simulink model "GuytonModel1986All_R2015a"  (R2015a)
settings: Solver=ode15s  StartTime=0  StopTime=383040  FixedStep=0.03  MaxStep=360  RelTol=1e-3
libraries: simulink x3
(part 5 of 5)

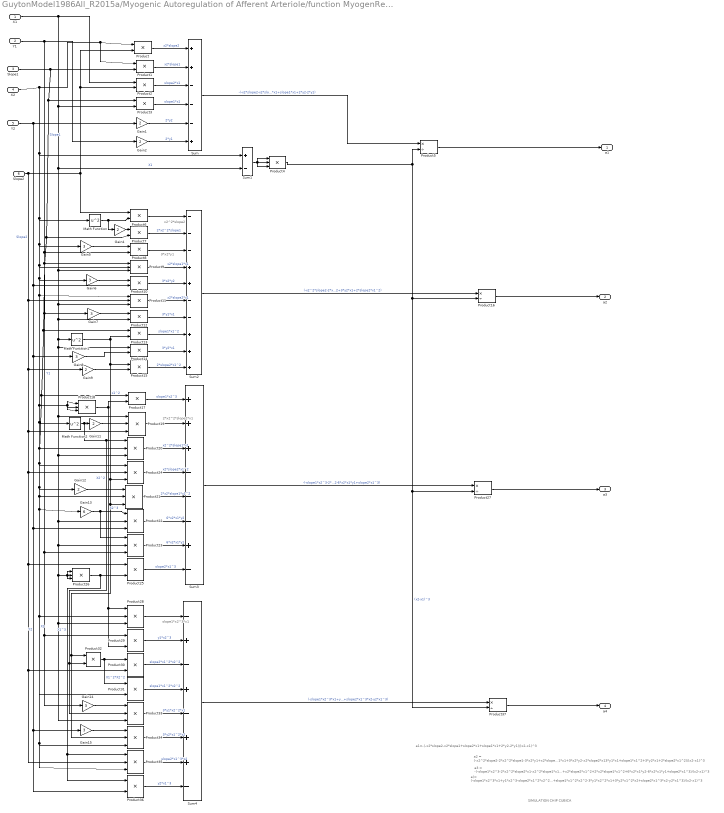
== system GuytonModel1986All_R2015a/Myogenic Autoregulation of Afferent Arteriole/function MyogenResp(PDIFF) - spline interpolation/If Action Subsystem/Cubica ==
  note: SIMULATION CHIP CUBICA
  note: a)= (-slope1*x2^3*x1+y1*x2^3-slope2*x1^2*x2^2+slope1*x1^2*x2^2-3*y1*x2^2*x1+3*y2*x1^2*x2+slope2*x1^3*x2-y2*x1^3)/(x2-x1)^3
  note: a3 = -(-slope1*x2^3-2*x2^2*slope2*x1-x2^2*slope1*x1+x2*slope2*x1^2+2*x2*slope1*x1^2+6*x2*x1*y2-6*x2*x1*y1+slope2*x1^3)/(x2-x1)^3
  note: a2 = (-x2^2*slope2-2*x2^2*slope1-3*x2*y1+x2*slope1*x1+3*x2*y2-x2*slope2*x13*y1*x1+slope1*x1^2+3*y2*x1+2*slope2*x1^2)/(x2-x1)^3
  note: slope1*x2^3*x1
  note: 2*x2^2*slope2*x1
  note: 3*x2*y1
  note: x2^2*slope2
  note: a1=-(-x2*slope2-x2*slope1+slope2*x1+slope1*x1+2*y2-2*y1)/(x2-x1)^3
  X1 : Inport
  Y1 : Inport  Port=2
  Slope1 : Inport  Port=3
  X2 : Inport  Port=4
  Y2 : Inport  Port=5
  Slope2 : Inport  Port=6
  Gain{1..2,4,9,11..12} (6 alike) : Gain  Gain=2  SaturateOnIntegerOverflow=on  OutDataTypeStr=Inherit: Same as input  ParamDataTypeStr=Inherit: Same as input
  Gain13 : Gain  Gain=6  SaturateOnIntegerOverflow=on  OutDataTypeStr=Inherit: Same as input  ParamDataTypeStr=Inherit: Same as input
  Gain{5..8,14..15} (6 alike) : Gain  Gain=3  SaturateOnIntegerOverflow=on  OutDataTypeStr=Inherit: Same as input  ParamDataTypeStr=Inherit: Same as input
  Math Function : Math  Operator=square  SaturateOnIntegerOverflow=on
  Math Function1 : Math  Operator=square  SaturateOnIntegerOverflow=on
  Math Function2 : Math  Operator=square  SaturateOnIntegerOverflow=on
  Product{,1..3,6..8,10,12..15,17,25,29..32,36} (19 alike) : Product  SaturateOnIntegerOverflow=on  InputSameDT=on  OutDataTypeStr=Inherit: Same as first input
  Product{4,9,11,18..24,26,28,33..35} (15 alike) : Product  Inputs=3  SaturateOnIntegerOverflow=on  InputSameDT=on  OutDataTypeStr=Inherit: Same as first input
  Product{5,16,27,37} (4 alike) : Product  Inputs=*/  SaturateOnIntegerOverflow=on  InputSameDT=on  OutDataTypeStr=Inherit: Same as first input
  Sum : Sum  Inputs=++---+  SaturateOnIntegerOverflow=on  InputSameDT=on  OutDataTypeStr=Inherit: Same as first input
  Sum1 : Sum  Inputs=+-  SaturateOnIntegerOverflow=on  InputSameDT=on  OutDataTypeStr=Inherit: Same as first input
  Sum2 : Sum  Inputs=---++--+++  SaturateOnIntegerOverflow=on  InputSameDT=on  OutDataTypeStr=Inherit: Same as first input
  Sum3 : Sum  Inputs=+++---+-  SaturateOnIntegerOverflow=on  InputSameDT=on  OutDataTypeStr=Inherit: Same as first input
  Sum4 : Sum  Inputs=-+-+-++-  SaturateOnIntegerOverflow=on  InputSameDT=on  OutDataTypeStr=Inherit: Same as first input
  a1 : Outport
  a2 : Outport  Port=2
  a3 : Outport  Port=3
  a4 : Outport  Port=4
  wires:
  Sum3/1 -> Product27/1  "-(-slope1*x2^3-2*x2^2*slope2*x1-x2^2*slope1*x1+x2*slope2*x1^2+2*x2*slope1*x1^2+6*x2*x1*y2-6*x2*x1*y1+slope2*x1^3)"
  Product37/1 -> a4/1
  Sum4/1 -> Product37/1  "(-slope1*x2^3*x1+y1*x2^3-slope2*x1^2*x2^2+slope1*x1^2*x2^2-3*y1*x2^2*x1+3*y2*x1^2*x2+slope2*x1^3*x2-y2*x1^3)"
  Product36/1 -> Sum4/8  "y2*x1^3"
  Product35/1 -> Sum4/7  "slope2*x1^3*x2"
  Gain15/1 -> Product34/1
  Product34/1 -> Sum4/6  "3*y2*x1^2*x2"
  Gain14/1 -> Product33/1
  Product33/1 -> Sum4/5  "3*y1*x2^2*x1"
  Product32/1 -> Product31/1, Product30/1  "X1^2*X2^2"
  Product31/1 -> Sum4/4  "slope1*x1^2*x2^2"
  Product30/1 -> Sum4/3  "slope2*x1^2*x2^2"
  Product29/1 -> Sum4/2  "y1*x2^3"
  Product28/1 -> Sum4/1
  Product27/1 -> a3/1
  Product26/1 -> Product36/1, Product35/1, Product25/2  "X1^3"
  Product25/1 -> Sum3/8  "slope2*x1^3"
  Product24/1 -> Sum3/4  "x2*slope2*x1^2"
  Product21/1 -> Sum3/5  "2*x2*slope1*x1^2"
  Product22/1 -> Sum3/6  "6*x2*x1*y2"
  Product23/1 -> Sum3/7  "6*x2*x1*y1"
  Gain13/1 -> Product23/1, Product22/1
  Gain12/1 -> Product21/1
  Product20/1 -> Sum3/3  "x2^2*slope1*x1"
  Gain11/1 -> Product19/2
  Math Function2/1 -> Product33/2, Product32/2, Product20/1, Gain11/1  "X2^2"
  Product19/1 -> Sum3/2
  Product18/1 -> Product29/2, Product28/1, Product17/2  "X2^3"
  Product17/1 -> Sum3/1  "slope1*x2^3"
  Product16/1 -> a2/1
  Sum2/1 -> Product16/1  "(-x2^2*slope2-2*x2^2*slope1-3*x2*y1+x2*slope1*x1+3*x2*y2-x2*slope2*x1-3*y1*x1+slope1*x1^2+3*y2*x1+2*slope2*x1^2)"
  Gain9/1 -> Product15/2
  Product15/1 -> Sum2/10  "2*slope2*x1^2"
  Gain8/1 -> Product14/2
  Product14/1 -> Sum2/9  "3*y2*x1"
  Math Function1/1 -> Product34/2, Product32/1, Product21/3, Product24/3, Product15/1, Product13/2  "x1^2"
  Product13/1 -> Sum2/8  "slope1*x1^2"
  Gain7/1 -> Product12/1
  Product12/1 -> Sum2/7  "3*y1*x1"
  Product11/1 -> Sum2/6  "x2*slope2*x1"
  Product10/1 -> Sum2/5  "3*x2*y2"
  Gain6/1 -> Product10/1
  Product9/1 -> Sum2/4  "x2*slope1*x1"
  Gain5/1 -> Product8/1
  Product8/1 -> Sum2/3
  Product7/1 -> Sum2/2  "2*x2^2*slope1"
  Gain4/1 -> Product7/1
  Product6/1 -> Sum2/1
  Math Function/1 -> Gain4/1, Product6/2
  Product5/1 -> a1/1
  Product4/1 -> Product37/2, Product27/2, Product16/2, Product5/2  "(x2-x1)^3"
  Sum1/1 -> Product4/1, Product4/3, Product4/2
  Sum/1 -> Product5/1  "-(-x2*slope2-x2*slope1+slope2*x1+slope1*x1+2*y2-2*y1)"
  Y1/1 -> Gain14/1, Product29/1, Product23/3, Gain7/1, Product8/2, Gain2/1  "Y1"
  Gain2/1 -> Sum/6  "2*y1"
  Gain1/1 -> Sum/5  "2*y2"
  Y2/1 -> Product36/2, Gain15/1, Product22/3, Gain8/1, Product10/2, Gain1/1  "Y2"
  Product3/1 -> Sum/4  "slope1*x1"
  Product2/1 -> Sum/3  "slope2*x1"
  X1/1 -> Sum1/2, Product33/3, Product28/3, Product26/1, Product26/3, Product26/2, Product23/2, Product22/2, Product20/3, Product19/1, Product14/1, Math Function1/1, Product12/2, Product11/3, Product9/3, Product3/2, Product2/1  "X1"
  Product1/1 -> Sum/2  "x2*slope1"
  Product/1 -> Sum/1  "x2*slope2"
  Slope1/1 -> Product31/2, Product28/2, Product21/2, Product20/2, Product17/1, Product13/1, Product9/1, Product7/2, Product3/1, Product1/2  "Slope1"
  Slope2/1 -> Product35/2, Product30/2, Product25/1, Product24/2, Product19/3, Gain9/1, Product11/2, Product6/1, Product2/2, Product/2  "Slope2"
  X2/1 -> Product/1, Product1/1, Product24/1, Product35/3, Product34/3, Gain13/1, Gain12/1, Math Function2/1, Product18/3, Product18/1, Product18/2, Product11/1, Gain6/1, Product9/2, Gain5/1, Math Function/1, Sum1/1  "X2"

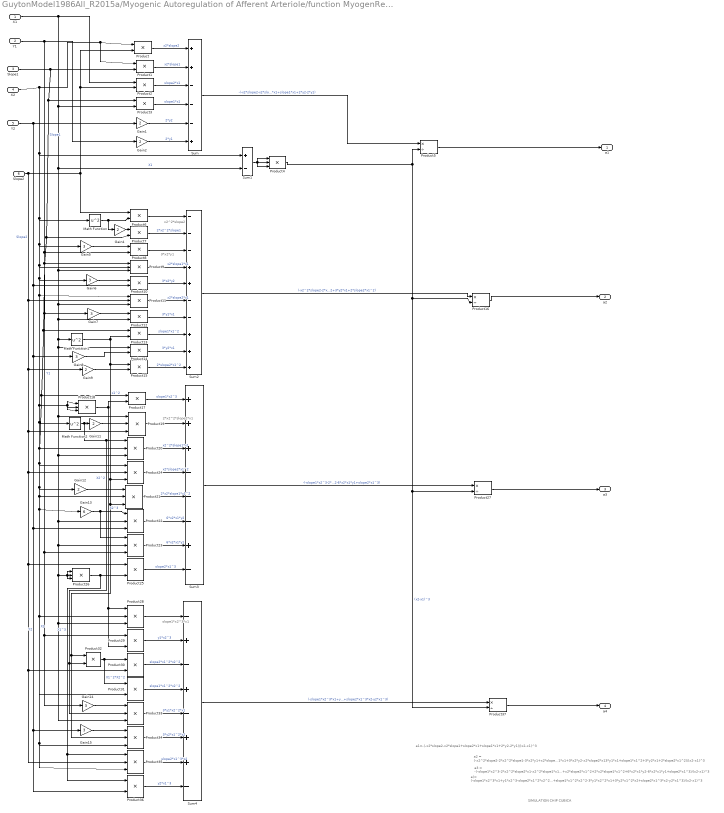
== system GuytonModel1986All_R2015a/Myogenic Autoregulation of Afferent Arteriole/function MyogenResp(PDIFF) - spline interpolation/If Action Subsystem/Cubica1 ==
  note: SIMULATION CHIP CUBICA
  note: a)= (-slope1*x2^3*x1+y1*x2^3-slope2*x1^2*x2^2+slope1*x1^2*x2^2-3*y1*x2^2*x1+3*y2*x1^2*x2+slope2*x1^3*x2-y2*x1^3)/(x2-x1)^3
  note: a3 = -(-slope1*x2^3-2*x2^2*slope2*x1-x2^2*slope1*x1+x2*slope2*x1^2+2*x2*slope1*x1^2+6*x2*x1*y2-6*x2*x1*y1+slope2*x1^3)/(x2-x1)^3
  note: a2 = (-x2^2*slope2-2*x2^2*slope1-3*x2*y1+x2*slope1*x1+3*x2*y2-x2*slope2*x13*y1*x1+slope1*x1^2+3*y2*x1+2*slope2*x1^2)/(x2-x1)^3
  note: slope1*x2^3*x1
  note: 2*x2^2*slope2*x1
  note: 3*x2*y1
  note: x2^2*slope2
  note: a1=-(-x2*slope2-x2*slope1+slope2*x1+slope1*x1+2*y2-2*y1)/(x2-x1)^3
  X1 : Inport
  Y1 : Inport  Port=2
  Slope1 : Inport  Port=3
  X2 : Inport  Port=4
  Y2 : Inport  Port=5
  Slope2 : Inport  Port=6
  Gain{1..2,4,9,11..12} (6 alike) : Gain  Gain=2  SaturateOnIntegerOverflow=on  OutDataTypeStr=Inherit: Same as input  ParamDataTypeStr=Inherit: Same as input
  Gain13 : Gain  Gain=6  SaturateOnIntegerOverflow=on  OutDataTypeStr=Inherit: Same as input  ParamDataTypeStr=Inherit: Same as input
  Gain{5..8,14..15} (6 alike) : Gain  Gain=3  SaturateOnIntegerOverflow=on  OutDataTypeStr=Inherit: Same as input  ParamDataTypeStr=Inherit: Same as input
  Math Function : Math  Operator=square  SaturateOnIntegerOverflow=on
  Math Function1 : Math  Operator=square  SaturateOnIntegerOverflow=on
  Math Function2 : Math  Operator=square  SaturateOnIntegerOverflow=on
  Product{,1..3,6..8,10,12..15,17,25,29..32,36} (19 alike) : Product  SaturateOnIntegerOverflow=on  InputSameDT=on  OutDataTypeStr=Inherit: Same as first input
  Product{4,9,11,18..24,26,28,33..35} (15 alike) : Product  Inputs=3  SaturateOnIntegerOverflow=on  InputSameDT=on  OutDataTypeStr=Inherit: Same as first input
  Product{5,16,27,37} (4 alike) : Product  Inputs=*/  SaturateOnIntegerOverflow=on  InputSameDT=on  OutDataTypeStr=Inherit: Same as first input
  Sum : Sum  Inputs=++---+  SaturateOnIntegerOverflow=on  InputSameDT=on  OutDataTypeStr=Inherit: Same as first input
  Sum1 : Sum  Inputs=+-  SaturateOnIntegerOverflow=on  InputSameDT=on  OutDataTypeStr=Inherit: Same as first input
  Sum2 : Sum  Inputs=---++--+++  SaturateOnIntegerOverflow=on  InputSameDT=on  OutDataTypeStr=Inherit: Same as first input
  Sum3 : Sum  Inputs=+++---+-  SaturateOnIntegerOverflow=on  InputSameDT=on  OutDataTypeStr=Inherit: Same as first input
  Sum4 : Sum  Inputs=-+-+-++-  SaturateOnIntegerOverflow=on  InputSameDT=on  OutDataTypeStr=Inherit: Same as first input
  a1 : Outport
  a2 : Outport  Port=2
  a3 : Outport  Port=3
  a4 : Outport  Port=4
  wires:
  Sum3/1 -> Product27/1  "-(-slope1*x2^3-2*x2^2*slope2*x1-x2^2*slope1*x1+x2*slope2*x1^2+2*x2*slope1*x1^2+6*x2*x1*y2-6*x2*x1*y1+slope2*x1^3)"
  Product37/1 -> a4/1
  Sum4/1 -> Product37/1  "(-slope1*x2^3*x1+y1*x2^3-slope2*x1^2*x2^2+slope1*x1^2*x2^2-3*y1*x2^2*x1+3*y2*x1^2*x2+slope2*x1^3*x2-y2*x1^3)"
  Product36/1 -> Sum4/8  "y2*x1^3"
  Product35/1 -> Sum4/7  "slope2*x1^3*x2"
  Gain15/1 -> Product34/1
  Product34/1 -> Sum4/6  "3*y2*x1^2*x2"
  Gain14/1 -> Product33/1
  Product33/1 -> Sum4/5  "3*y1*x2^2*x1"
  Product32/1 -> Product31/1, Product30/1  "X1^2*X2^2"
  Product31/1 -> Sum4/4  "slope1*x1^2*x2^2"
  Product30/1 -> Sum4/3  "slope2*x1^2*x2^2"
  Product29/1 -> Sum4/2  "y1*x2^3"
  Product28/1 -> Sum4/1
  Product27/1 -> a3/1
  Product26/1 -> Product36/1, Product35/1, Product25/2  "X1^3"
  Product25/1 -> Sum3/8  "slope2*x1^3"
  Product24/1 -> Sum3/4  "x2*slope2*x1^2"
  Product21/1 -> Sum3/5  "2*x2*slope1*x1^2"
  Product22/1 -> Sum3/6  "6*x2*x1*y2"
  Product23/1 -> Sum3/7  "6*x2*x1*y1"
  Gain13/1 -> Product23/1, Product22/1
  Gain12/1 -> Product21/1
  Product20/1 -> Sum3/3  "x2^2*slope1*x1"
  Gain11/1 -> Product19/2
  Math Function2/1 -> Product33/2, Product32/2, Product20/1, Gain11/1  "X2^2"
  Product19/1 -> Sum3/2
  Product18/1 -> Product29/2, Product28/1, Product17/2  "X2^3"
  Product17/1 -> Sum3/1  "slope1*x2^3"
  Product16/1 -> a2/1
  Sum2/1 -> Product16/1  "(-x2^2*slope2-2*x2^2*slope1-3*x2*y1+x2*slope1*x1+3*x2*y2-x2*slope2*x1-3*y1*x1+slope1*x1^2+3*y2*x1+2*slope2*x1^2)"
  Gain9/1 -> Product15/2
  Product15/1 -> Sum2/10  "2*slope2*x1^2"
  Gain8/1 -> Product14/2
  Product14/1 -> Sum2/9  "3*y2*x1"
  Math Function1/1 -> Product34/2, Product32/1, Product21/3, Product24/3, Product15/1, Product13/2  "x1^2"
  Product13/1 -> Sum2/8  "slope1*x1^2"
  Gain7/1 -> Product12/1
  Product12/1 -> Sum2/7  "3*y1*x1"
  Product11/1 -> Sum2/6  "x2*slope2*x1"
  Product10/1 -> Sum2/5  "3*x2*y2"
  Gain6/1 -> Product10/1
  Product9/1 -> Sum2/4  "x2*slope1*x1"
  Gain5/1 -> Product8/1
  Product8/1 -> Sum2/3
  Product7/1 -> Sum2/2  "2*x2^2*slope1"
  Gain4/1 -> Product7/1
  Product6/1 -> Sum2/1
  Math Function/1 -> Gain4/1, Product6/2
  Product5/1 -> a1/1
  Product4/1 -> Product37/2, Product27/2, Product16/2, Product5/2  "(x2-x1)^3"
  Sum1/1 -> Product4/1, Product4/3, Product4/2
  Sum/1 -> Product5/1  "-(-x2*slope2-x2*slope1+slope2*x1+slope1*x1+2*y2-2*y1)"
  Y1/1 -> Gain14/1, Product29/1, Product23/3, Gain7/1, Product8/2, Gain2/1  "Y1"
  Gain2/1 -> Sum/6  "2*y1"
  Gain1/1 -> Sum/5  "2*y2"
  Y2/1 -> Product36/2, Gain15/1, Product22/3, Gain8/1, Product10/2, Gain1/1  "Y2"
  Product3/1 -> Sum/4  "slope1*x1"
  Product2/1 -> Sum/3  "slope2*x1"
  X1/1 -> Sum1/2, Product33/3, Product28/3, Product26/1, Product26/3, Product26/2, Product23/2, Product22/2, Product20/3, Product19/1, Product14/1, Math Function1/1, Product12/2, Product11/3, Product9/3, Product3/2, Product2/1  "X1"
  Product1/1 -> Sum/2  "x2*slope1"
  Product/1 -> Sum/1  "x2*slope2"
  Slope1/1 -> Product31/2, Product28/2, Product21/2, Product20/2, Product17/1, Product13/1, Product9/1, Product7/2, Product3/1, Product1/2  "Slope1"
  Slope2/1 -> Product35/2, Product30/2, Product25/1, Product24/2, Product19/3, Gain9/1, Product11/2, Product6/1, Product2/2, Product/2  "Slope2"
  X2/1 -> Product/1, Product1/1, Product24/1, Product35/3, Product34/3, Gain13/1, Gain12/1, Math Function2/1, Product18/3, Product18/1, Product18/2, Product11/1, Gain6/1, Product9/2, Gain5/1, Math Function/1, Sum1/1  "X2"

== system GuytonModel1986All_R2015a/Myogenic Autoregulation of Afferent Arteriole/function MyogenResp(PDIFF) - spline interpolation/Subsystem/If Action Subsystem ==
  x : Inport
  aa4 : Inport  Port=2
  "aa6 " : Inport  Port=3
  Action Port : ActionPort  ActionType=then
  Product : Product  SaturateOnIntegerOverflow=on  InputSameDT=on  OutDataTypeStr=Inherit: Same as first input
  Sum : Sum  SaturateOnIntegerOverflow=on  InputSameDT=on  OutDataTypeStr=Inherit: Same as first input
  y : Outport
  wires:
  Sum/1 -> y/1  "y=aa4*x+aa5"
  "aa6 "/1 -> Sum/2
  Product/1 -> Sum/1
  x/1 -> Product/1
  aa4/1 -> Product/2

== system GuytonModel1986All_R2015a/Myogenic Autoregulation of Afferent Arteriole/function MyogenResp(PDIFF) - spline interpolation/Subsystem/If Action Subsystem1 ==
  x : Inport
  aa6 : Inport  Port=2
  aa7 : Inport  Port=3
  aa8 : Inport  Port=4
  aa9 : Inport  Port=5
  Action Port : ActionPort  ActionType=elseif
  Math Function : Math  Operator=square  SaturateOnIntegerOverflow=on
  Product : Product  Inputs=3  SaturateOnIntegerOverflow=on  InputSameDT=on  OutDataTypeStr=Inherit: Same as first input
  Product2 : Product  SaturateOnIntegerOverflow=on  InputSameDT=on  OutDataTypeStr=Inherit: Same as first input
  Product3 : Product  SaturateOnIntegerOverflow=on  InputSameDT=on  OutDataTypeStr=Inherit: Same as first input
  Sum : Sum  Inputs=++++  SaturateOnIntegerOverflow=on  InputSameDT=on  OutDataTypeStr=Inherit: Same as first input
  y : Outport
  wires:
  Sum/1 -> y/1  "y=aa6*x^3+aa7*x^2+aa8*x+aa9"
  aa9/1 -> Sum/4
  Product3/1 -> Sum/3
  aa8/1 -> Product3/2
  Product2/1 -> Sum/2
  aa7/1 -> Product2/2
  aa6/1 -> Product/3
  Product/1 -> Sum/1
  Math Function/1 -> Product2/1, Product/1
  x/1 -> Product3/1, Product/2, Math Function/1

== system GuytonModel1986All_R2015a/Myogenic Autoregulation of Afferent Arteriole/function MyogenResp(PDIFF) - spline interpolation/Subsystem/If Action Subsystem2 ==
  x : Inport
  aa10 : Inport  Port=2
  aa11 : Inport  Port=3
  aa12 : Inport  Port=4
  aa13 : Inport  Port=5
  Action Port : ActionPort  ActionType=elseif
  Math Function : Math  Operator=square  SaturateOnIntegerOverflow=on
  Product : Product  Inputs=3  SaturateOnIntegerOverflow=on  InputSameDT=on  OutDataTypeStr=Inherit: Same as first input
  Product2 : Product  SaturateOnIntegerOverflow=on  InputSameDT=on  OutDataTypeStr=Inherit: Same as first input
  Product3 : Product  SaturateOnIntegerOverflow=on  InputSameDT=on  OutDataTypeStr=Inherit: Same as first input
  Sum : Sum  Inputs=++++  SaturateOnIntegerOverflow=on  InputSameDT=on  OutDataTypeStr=Inherit: Same as first input
  y : Outport
  wires:
  x/1 -> Math Function/1, Product/2, Product3/1
  Math Function/1 -> Product/1, Product2/1
  Product/1 -> Sum/1
  aa10/1 -> Product/3
  aa11/1 -> Product2/2
  Product2/1 -> Sum/2
  aa12/1 -> Product3/2
  Product3/1 -> Sum/3
  aa13/1 -> Sum/4
  Sum/1 -> y/1  "y=aa6*x^3+aa7*x^2+aa8*x+aa9"

== system GuytonModel1986All_R2015a/Myogenic Autoregulation of Afferent Arteriole/function MyogenResp(PDIFF) - spline interpolation/Subsystem/If Action Subsystem3 ==
  x : Inport
  aa14 : Inport  Port=2
  aa15 : Inport  Port=3
  Action Port : ActionPort  ActionType=else
  Product3 : Product  SaturateOnIntegerOverflow=on  InputSameDT=on  OutDataTypeStr=Inherit: Same as first input
  Sum : Sum  SaturateOnIntegerOverflow=on  InputSameDT=on  OutDataTypeStr=Inherit: Same as first input
  Out1 : Outport
  wires:
  Sum/1 -> Out1/1
  Product3/1 -> Sum/1
  aa15/1 -> Sum/2
  x/1 -> Product3/1
  aa14/1 -> Product3/2
